simulink model "CurrentController_TestHarness"  (R2017b)
settings: Solver=VariableStepAuto  StartTime=0.0  StopTime=2  RelTol=1e-3
undefined symbols (not defined in the file): DiscIntNeverNeededParam, Kp_cc, Lf, Rf, Ts, wn
settings Model: Creator=saioa  LastModifiedBy=saioa

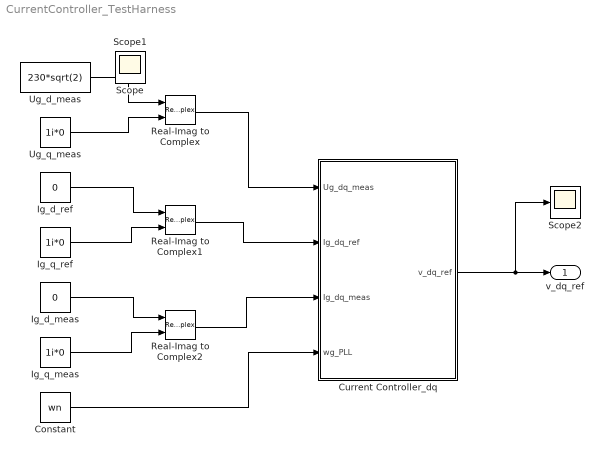
== system CurrentController_TestHarness ==
  Constant : Constant  Value=wn
  Current Controller_dq : Subsystem
  Ig_d_meas : Constant  Value=0
  Ig_d_ref : Constant  Value=0
  Ig_q_meas : Constant  Value=1i*0
  Ig_q_ref : Constant  Value=1i*0
  Real-Imag to Complex : RealImagToComplex
  Real-Imag to Complex1 : RealImagToComplex
  Real-Imag to Complex2 : RealImagToComplex
  Scope2 : Scope
  Ug_d_meas : Constant  Value=230*sqrt(2)
  Ug_q_meas : Constant  Value=1i*0
  v_dq_ref : Outport
  Scope : Scope
  Scope1 : Scope
  wires:
  Real-Imag to Complex2/1 -> Current Controller_dq/3(Ig_dq_meas)
  Real-Imag to Complex1/1 -> Current Controller_dq/2(Ig_dq_ref)
  Current Controller_dq/1(v_dq_ref) -> Scope2/1, v_dq_ref/1
  Real-Imag to Complex/1 -> Current Controller_dq/1(Ug_dq_meas)
  Ug_d_meas/1 -> Real-Imag to Complex/1
  Ug_q_meas/1 -> Real-Imag to Complex/2
  Ig_d_ref/1 -> Real-Imag to Complex1/1
  Ig_q_ref/1 -> Real-Imag to Complex1/2
  Ig_d_meas/1 -> Real-Imag to Complex2/1
  Ig_q_meas/1 -> Real-Imag to Complex2/2
  Constant/1 -> Current Controller_dq/4(wg_PLL)

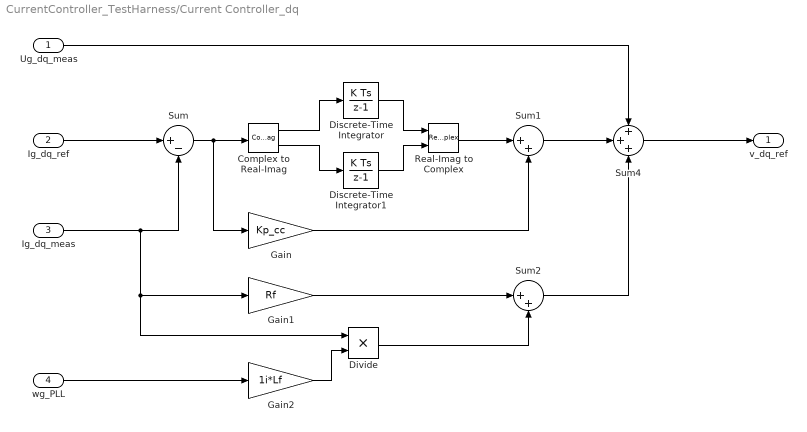
== system CurrentController_TestHarness/Current Controller_dq ==
  Ug_dq_meas : Inport
  Ig_dq_ref : Inport  Port=2
  Ig_dq_meas : Inport  Port=3
  wg_PLL : Inport  Port=4
  Complex to Real-Imag : ComplexToRealImag
  Discrete-Time Integrator : DiscreteIntegrator  gainval=Ki_cc  InitialConditionSetting=State (most efficient)  SampleTime=Ts  ICPrevOutput=DiscIntNeverNeededParam  ICPrevScaledInput=DiscIntNeverNeededParam
  Discrete-Time Integrator1 : DiscreteIntegrator  gainval=Ki_cc  InitialConditionSetting=State (most efficient)  SampleTime=Ts  ICPrevOutput=DiscIntNeverNeededParam  ICPrevScaledInput=DiscIntNeverNeededParam
  Divide : Product  Inputs=**
  Gain : Gain  Gain=Kp_cc
  Gain1 : Gain  Gain=Rf
  Gain2 : Gain  Gain=1i*Lf
  Real-Imag to Complex : RealImagToComplex
  Sum : Sum  Inputs=|+-
  Sum1 : Sum  Inputs=|++
  Sum2 : Sum  Inputs=|++
  Sum4 : Sum  Inputs=+++  SaturateOnIntegerOverflow=on  InputSameDT=on  OutDataTypeStr=Inherit: Same as first input
  v_dq_ref : Outport
  wires:
  Ig_dq_meas/1 -> Gain1/1, Divide/1, Sum/2
  Sum/1 -> Gain/1, Complex to Real-Imag/1
  Ig_dq_ref/1 -> Sum/1
  Discrete-Time Integrator1/1 -> Real-Imag to Complex/2
  wg_PLL/1 -> Gain2/1
  Gain/1 -> Sum1/2
  Complex to Real-Imag/2 -> Discrete-Time Integrator1/1
  Discrete-Time Integrator/1 -> Real-Imag to Complex/1
  Real-Imag to Complex/1 -> Sum1/1
  Complex to Real-Imag/1 -> Discrete-Time Integrator/1
  Sum1/1 -> Sum4/2
  Sum2/1 -> Sum4/3
  Divide/1 -> Sum2/2
  Ug_dq_meas/1 -> Sum4/1
  Sum4/1 -> v_dq_ref/1
  Gain2/1 -> Divide/2
  Gain1/1 -> Sum2/1
